simulink model "proj2_week2_new"  (R2021a)
settings: Solver=VariableStepAuto  StartTime=0.0  StopTime=10.0  RelTol=1e-3
model workspace (MAT data in the model file):
  b = Simulink.Parameter
  b.Value = 50
  b.DataType = 'auto'
  b.Dimensions = [1 1]
  k1 = Simulink.Parameter
  k1.Value = 50
  k1.DataType = 'auto'
  k1.Dimensions = [1 1]
  k2 = Simulink.Parameter
  k2.Value = 60
  k2.DataType = 'auto'
  k2.Dimensions = [1 1]
  m1 = Simulink.Parameter
  m1.Value = 100
  m1.DataType = 'auto'
  m1.Dimensions = [1 1]
  m2 = Simulink.Parameter
  m2.Value = 50
  m2.DataType = 'auto'
  m2.Dimensions = [1 1]
settings Model: Creator=RASIKA MALGI  LastModifiedBy=RASIKA MALGI

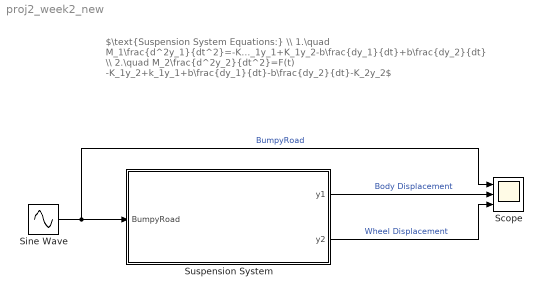
== system proj2_week2_new ==
  note: $\text{Suspension System Equations:} \\ 1.\quad M_1\frac{d^2y_1}{dt^2}=-K_1y_1+K_1y_2-b\frac{dy_1}{dt}+b\frac{dy_2}{dt} \\ 2.\quad M_2\frac{d^2y_2}{dt^2}=F(t) -K_1y_2+k_1y_1+b\frac{dy_1}{dt}-b\frac{dy_2}{dt}-K_2y_2$
  Scope : Scope  NumInputPorts=3
  Sine Wave : Sin  SampleTime=0
  Suspension System : Subsystem
  wires:
  Sine Wave/1 -> Scope/1, Suspension System/1(BumpyRoad)  "BumpyRoad"
  Suspension System/2(y2) -> Scope/3  "Wheel Displacement"
  Suspension System/1(y1) -> Scope/2  "Body Displacement"

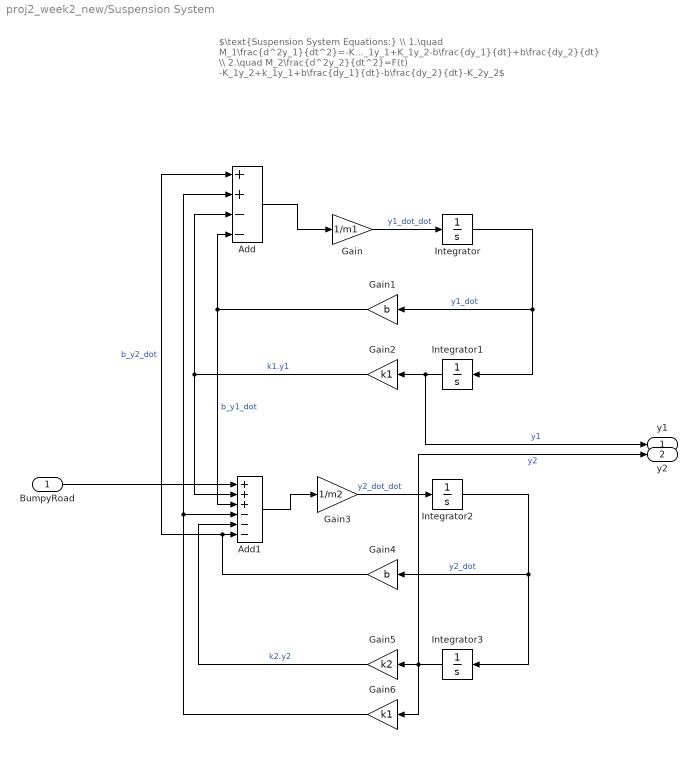
== system proj2_week2_new/Suspension System ==
  note: $\text{Suspension System Equations:} \\ 1.\quad M_1\frac{d^2y_1}{dt^2}=-K_1y_1+K_1y_2-b\frac{dy_1}{dt}+b\frac{dy_2}{dt} \\ 2.\quad M_2\frac{d^2y_2}{dt^2}=F(t) -K_1y_2+k_1y_1+b\frac{dy_1}{dt}-b\frac{dy_2}{dt}-K_2y_2$
  BumpyRoad : Inport
  Add : Sum  Inputs=++--
  Add1 : Sum  Inputs=+++---
  Gain : Gain  Gain=1/m1
  Gain1 : Gain  Gain=b
  Gain2 : Gain  Gain=k1
  Gain3 : Gain  Gain=1/m2
  Gain4 : Gain  Gain=b
  Gain5 : Gain  Gain=k2
  Gain6 : Gain  Gain=k1
  Integrator{,1..3} (4 alike) : Integrator
  y1 : Outport
  y2 : Outport  Port=2
  wires:
  Integrator/1 -> Integrator1/1, Gain1/1  "y1_dot"
  Gain5/1 -> Add1/5  "k2.y2"
  Add/1 -> Gain/1
  Gain/1 -> Integrator/1  "y1_dot_dot"
  Gain1/1 -> Add/4, Add1/3  "b_y1_dot"
  Gain4/1 -> Add/1, Add1/6  "b_y2_dot"
  Add1/1 -> Gain3/1
  Integrator2/1 -> Integrator3/1, Gain4/1  "y2_dot"
  Integrator1/1 -> y1/1, Gain2/1  "y1"
  Gain2/1 -> Add1/2, Add/3  "k1.y1"
  Gain6/1 -> Add/2, Add1/4
  Gain3/1 -> Integrator2/1  "y2_dot_dot"
  Integrator3/1 -> y2/1, Gain6/1, Gain5/1  "y2"
  BumpyRoad/1 -> Add1/1
